simulink model "Milford"  (R2017a)
settings: Solver=FixedStepAuto  StartTime=0.0  StopTime=Cycle_End  FixedStep=0.01  MaxStep=0.01  RelTol=1e-3  EnableMultiTasking=on
PostLoadFcn:
  | , if any(exist('dsrtsu_mdlpostloadfcn', 'file') == [2, 3, 6]), try dsrtsu_mdlpostloadfcn('Execute', bdroot); catch fprintf('Error in PostLoadFcn (dsrtsu_mdlpostloadfcn) for model "%s":\n %s\n', bdroot, lasterr); end, end,
undefined symbols (not defined in the file): Actuators, APP1_OOR, APP2_OOR, APP_Mismatch, Brk_Flt, cal, ClutchEngag, DiscIntNeverNeededParam, eng, Engine, EngOverTemp, ENGTRQ_MSMCH_Degraded_CP, ENGTRQ_MSMCH_ErrCritical_CP, ENGTRQ_MSMCH_LimpHome_CP, EngTrqMismatch, ESSOverTemp, gb, Gearbox, KeyPos_Flt, lib_Actuators, lib_Sensors_2017a, lib_Transmission, Loss, LossCAN, MCUOverTemp, mot, MotDirMismatch, MotOverTemp, MotTrqMismatch, mph2kph, PRNDL_Flt, Ratio, RegenFault, Sensors, Spd, time, Transmission
libraries: simulink x110, powerlib_meascontrol x6, EC2_libraries x5, dspsigops x3, lib_Chassis x1, lib_DCDC x1, lib_Differential x1, lib_HVESS x1, lib_Engine x1, lib_OBC x1, Transmission_Validation x1, lib_Wheels x1
(part 4 of 9)

== system Milford/Controller_with_Transmission_Manager1/HSC/Driver_Requests/APP_BPP to DrvIntndAxlTrq2/Post Driver Intnded Axle Torque ==
  note: //*mode==1 (CD Mode)
      | mode==2 (CS Mode - Engine Drive)
      | mode==3 (CS Mode-Motor Drive) pass MotTrq
      | mode==4 (Sports Mode) pass Mot Trq+Eng Trq
      | mode==5 (Engine only mode)*//
  APP : Inport
  BPP : Inport  Port=2
  VehicleSpeed : Inport  Port=3
  TransGearRatio : Inport  Port=4
  Mode : Inport  Port=5
  Motor_Speed : Inport  Port=6
  APP1 : InportShadow
  Abs : Abs
  Add : Sum
  Brake Command : Subsystem
  Bus Creator1 : BusCreator  Inputs=1
  Bus Creator3 : BusCreator  Inputs=3
  Driver Intended Axle Torque : Subsystem
  Switch : Switch  Threshold=cal.Regen.MinMotSpd
  rad/s to RPM2 : Gain  Gain=30/pi
  IntndAxlTrq : Outport
  BrkIntndAxlTrq : Outport  Port=2
  tag scope: DrvIntdAxleTrq=global
  wires:
  APP/1 -> Brake Command/1(APP)
  Driver Intended Axle Torque/1(DrvIntndAxlTrq) -> Add/1, [DrvIntdAxleTrq]  "DrvIntndAxlTrq"
  BPP/1 -> Brake Command/2(BPP)
  VehicleSpeed/1 -> Brake Command/3(VehicleSpeed)
  Mode/1 -> Driver Intended Axle Torque/2(Mode)
  TransGearRatio/1 -> Driver Intended Axle Torque/3(TransGearRatio)
  Brake Command/1(BrkAxlTrq) -> Add/2, Bus Creator1/1, Bus Creator3/3  "BrkIntndAxlTrq"
  Bus Creator1/1 -> BrkIntndAxlTrq/1
  Motor_Speed/1 -> rad/s to RPM2/1
  Abs/1 -> Switch/2
  Add/1 -> Switch/1  "FullDrvIntndAxlTrq"
  Switch/1 -> Bus Creator3/1  "FullDrvIntndAxlTrq"
  Bus Creator3/1 -> IntndAxlTrq/1  "IntndAxlTrq"
  [DrvIntdAxleTrq] -> Bus Creator3/2
  APP1/1 -> Driver Intended Axle Torque/1(APP)
  [DrvIntdAxleTrq] -> Switch/3
  rad/s to RPM2/1 -> Abs/1

== system Milford/Controller_with_Transmission_Manager1/HSC/Powertrain Manager/HV Manager/Axiomatic_Output_Manager ==
  Sensors : Inport
  HV_Bus_Status : Inport  Port=2
  Bus Creator : BusCreator  Inputs=3
  Bus Selector : BusSelector  OutputSignals=GFD_Light
  Bus Selector1 : BusSelector  OutputSignals=from_CAN.fromHV_CAN.from_OBC.NLG5_ST.NLG5_S_CP_DT,from_CAN.fromEBCAN.from_ECM.EngRunAtv
  Compare To Constant1 : simulink/Logic and Bit Operations/Compare To Constant  relop===  const=1  OutDataTypeStr=boolean
  Data Type Conversion : DataTypeConversion
  Logical Operator : Logic  AllPortsSameDT=off  OutDataTypeStr=boolean
  Logical Operator1 : Logic  Operator=NOT  AllPortsSameDT=off  OutDataTypeStr=boolean
  Axiomatic_CAN : Outport
  wires:
  [HV_Charge_Indicator] -> Data Type Conversion/1
  Sensors/1 -> Bus Selector1/1
  Logical Operator/1 -> Bus Creator/3  "Veh_Ready_Light"
  Data Type Conversion/1 -> Bus Creator/2  "HV_Chg_Light"
  Bus Selector/1 -> Bus Creator/1  "<GFD_Light>"
  Bus Creator/1 -> Axiomatic_CAN/1  "Axiomatic_CAN"
  HV_Bus_Status/1 -> Bus Selector/1
  Compare To Constant1/1 -> Logical Operator/2
  Logical Operator1/1 -> Logical Operator/1
  Bus Selector1/2 -> Compare To Constant1/1  "<EngRunAtv>"
  Bus Selector1/1 -> Logical Operator1/1  "<NLG5_S_CP_DT>"

== system Milford/Controller_with_Transmission_Manager1/HSC/Powertrain Manager/HV Manager/BMS_Manager ==
  note: Control Pilot signal added 02/14/2017
      | to charge automatically
  Sensors : Inport
  Controls : Inport  Port=2
  Bus Creator : BusCreator  Inputs=3
  Bus Creator1 : BusCreator  Inputs=8
  Bus Creator2 : BusCreator  Inputs=2
  Bus Creator3 : BusCreator  Inputs=6
  Bus Creator4 : BusCreator  Inputs=5
  Bus Selector : BusSelector  OutputSignals=closeMaincReq
  Bus Selector1 : BusSelector  OutputSignals=from_CAN.fromHV_CAN.from_BMSHybrid.BMS_HYB_02.BMS_Fehler_HS_offen,from_CAN.fromHV_CAN.from_BMSHybrid.BMS_HYB_02.BMS_Fehler_Pilot,from_CAN.fromHV_CAN.from_BMSHybrid.BMS_HYB_02.BMS_Init_abgeschlossen,from_CAN.fromHV_CAN.from_BMSHybrid.BMS_HYB_02.BMS_IstModus,from_CAN.fromHV_CAN.from_BMSHybrid.BMS_HYB_02.BMS_IstSpannung,from_CAN.fromHV_CAN.from_BMSHybrid.BMS_HYB_02.BMS_IstStrom,from_CAN.fromHV_CAN.from_BMSHybrid.BMS_HYB_02.BMS_SleepInd
  Bus Selector2 : BusSelector  OutputSignals=from_CAN.fromEBCAN.from_BMSAntrieb.NMH_BMS.NMH_BMS_Car_WakeUp,from_CAN.fromEBCAN.from_BMSAntrieb.NMH_BMS.NMH_BMS_Normal_Mode_1,from_CAN.fromEBCAN.from_BMSAntrieb.NMH_BMS.NMH_BMS_Normal_Mode_2,from_CAN.fromEBCAN.from_BMSAntrieb.NMH_BMS.NMH_BMS_Start_1,from_CAN.fromEBCAN.from_BMSAntrieb.NMH_BMS.NMH_BMS_Start_2,from_CAN.fromVEH_CAN.from_BCM.SysPwrMd,from_CAN.fromEBCAN.from_ECM.EngRunAtv
  Bus Selector3 : BusSelector  OutputSignals=from_CAN.fromHV_CAN.from_BMSHybrid.BMS_Spannung_ZwKr
  Bus Selector4 : BusSelector  OutputSignals=HV_req
  Bus Selector5 : BusSelector  OutputSignals=from_CAN.fromHV_CAN.from_OBC.NLG5_ST.NLG5_S_CP_DT
  Controls1 : InportShadow  Port=2
  Data Type Conversion{,1,6..8} (5 alike) : DataTypeConversion  OutDataTypeStr=boolean
  ESS_Manager : Stateflow chart  TreatAsAtomicUnit=on
  Edge Detector : powerlib_meascontrol/Logic/Edge Detector  model=Either  ic=0  Ts=0
      settings: SourceProductName=Simscape Power Systems  SourceProductBaseCode=PS
  Fault Latch : Subsystem
  ISO_Hybrid_01_Req : Subsystem
  Isolation Fault Calculation : Subsystem
  BMS CAN : Outport
  HV_BUS_Status : Outport  Port=2
  BMS Digital : Outport  Port=3
  wires:
  ISO_Hybrid_01_Req/1(Out1) -> Bus Creator/2
  ESS_Manager/9(ISO_Hybrid_01_Req) -> ISO_Hybrid_01_Req/1(In1)
  ESS_Manager/11(MO_BMS_Sollmodus) -> Bus Creator2/2
  Sensors/1 -> Bus Selector2/1, Bus Selector3/1, Isolation Fault Calculation/1(Sensors1), Bus Selector5/1, Bus Selector1/1
  Data Type Conversion1/1 -> Bus Creator4/5  "chg_wake"
  Bus Creator4/1 -> BMS Digital/1  "BMS_Digital"
  Bus Creator/1 -> BMS CAN/1  "BMS_CAN"
  Controls1/1 -> Bus Selector4/1
  Bus Selector/1 -> ESS_Manager/19(closeMaincReq)  "<closeMaincReq>"
  Controls/1 -> Bus Selector/1
  Bus Creator3/1 -> HV_BUS_Status/1  "HV_BUS_Status"
  ESS_Manager/18(HV_State) -> Bus Creator3/2
  ESS_Manager/15(veh_wake) -> Bus Creator4/4
  ESS_Manager/14(T_30C) -> Bus Creator4/3
  ESS_Manager/16(chga_wake) -> Data Type Conversion1/1
  ESS_Manager/13(T_30) -> Bus Creator4/2
  ESS_Manager/21(Shutdown_Complete) -> Bus Creator3/5
  ESS_Manager/20(ReadyToCharge) -> Data Type Conversion7/1
  ESS_Manager/19(ReadyToDrive) -> Data Type Conversion6/1
  ESS_Manager/17(HVDischarge) -> Data Type Conversion8/1
  Bus Creator1/1 -> Bus Creator/1  "ISO_Funktionaler_Req_All"
  Data Type Conversion8/1 -> Bus Creator3/1  "HV Discharge"
  Data Type Conversion7/1 -> Bus Creator3/4  "ReadyToCharge"
  Data Type Conversion6/1 -> Bus Creator3/3  "ReadyToDrive"
  ESS_Manager/12(T_15) -> Bus Creator4/1
  ESS_Manager/10(MO_SleepAckn) -> Bus Creator2/1
  ESS_Manager/8(Diag_Rq_Fktnl_Data_OBD_byte_7) -> Bus Creator1/8
  ESS_Manager/7(Diag_Rq_Fktnl_Data_OBD_byte_6) -> Bus Creator1/7
  ESS_Manager/6(Diag_Rq_Fktnl_Data_OBD_byte_5) -> Bus Creator1/6
  ESS_Manager/5(Diag_Rq_Fktnl_Data_OBD_byte_4) -> Bus Creator1/5
  ESS_Manager/4(Diag_Rq_Fktnl_Data_OBD_byte_3) -> Bus Creator1/4
  ESS_Manager/3(Diag_Rq_Fktnl_Data_OBD_byte_2) -> Bus Creator1/3
  ESS_Manager/2(Diag_Rq_Fktnl_Data_OBD_byte_1) -> Bus Creator1/2
  ESS_Manager/1(Diag_Rq_Fktnl_Data_OBD_byte_0) -> Bus Creator1/1
  Bus Selector5/1 -> Data Type Conversion/1  "<NLG5_S_CP_DT>"
  Bus Selector3/1 -> ESS_Manager/11(BMS_Spannung_ZwKr)  "<BMS_Spannung_ZwKr>"
  Bus Selector2/3 -> ESS_Manager/14(NMH_BMS_Normal_Mode_2)  "<NMH_BMS_Normal_Mode_2>"
  Bus Selector2/2 -> ESS_Manager/13(NMH_Normal_Mode_1)  "<NMH_BMS_Normal_Mode_1>"
  Bus Selector2/1 -> ESS_Manager/12(NMH_BMS_Car_WakeUp)  "<NMH_BMS_Car_WakeUp>"
  Bus Selector1/5 -> ESS_Manager/7(BMS_IstSpannung)  "<BMS_IstSpannung>"
  Bus Selector1/4 -> ESS_Manager/6(BMS_IstModus)  "<BMS_IstModus>"
  Bus Selector1/3 -> ESS_Manager/5(BMS_Init_abgeschlossen)  "<BMS_Init_abgeschlossen>"
  Bus Selector1/2 -> ESS_Manager/4(BMS_Fehler_Pilot)  "<BMS_Fehler_Pilot>"
  Bus Selector1/1 -> ESS_Manager/3(BMS_Fehler_HS_offen)  "<BMS_Fehler_HS_offen>"
  Isolation Fault Calculation/1(IsoFault) -> Fault Latch/1(IsoFault)
  Fault Latch/1(IsoFaultLatched) -> ESS_Manager/1(ISOfault)
  Bus Creator2/1 -> Bus Creator/3  "MSG_HYB_01"
  Bus Selector4/1 -> ESS_Manager/10(HV_req)  "<HV_req>"
  Bus Selector2/6 -> Edge Detector/1  "<SysPwrMd>"
  Edge Detector/1 -> ESS_Manager/17(KeyPos)
  Bus Selector2/7 -> ESS_Manager/18(EngRunAtv)  "<EngRunAtv>"
  Bus Selector2/5 -> ESS_Manager/16(NMH_BMS_Start_2)  "<NMH_BMS_Start_2>"
  Bus Selector2/4 -> ESS_Manager/15(NMH_BMS_Start_1)  "<NMH_BMS_Start_1>"
  Bus Selector1/7 -> ESS_Manager/9(BMS_SleepInd)  "<BMS_SleepInd>"
  Bus Selector1/6 -> ESS_Manager/8(BMS_IstStrom)  "<BMS_IstStrom>"
  Data Type Conversion/1 -> ESS_Manager/2(plugged)
  ESS_Manager/22(GFD_Light) -> Bus Creator3/6  "GFD_Light"

== system Milford/Controller_with_Transmission_Manager1/HSC/Powertrain Manager/HV Manager/DCDC Manager ==
  BMSInput : Inport
  Control : Inport  Port=2
  Bus Creator : BusCreator  Inputs=6
  Bus Selector : BusSelector  OutputSignals=from_CAN.fromHV_CAN.from_MCU.INV_VCU_01.INV_State
  Bus Selector1 : BusSelector  OutputSignals=from_CAN.fromHV_CAN.from_BMSHybrid.BMS_HYB_02.BMS_IstSpannung,from_CAN.fromHV_CAN.from_BMSHybrid.BMS_Spannung_ZwKr,from_CAN.fromHV_CAN.from_BMSHybrid.BMS_HYB_02.BMS_Fehler_Pilot
  Bus Selector2 : BusSelector  OutputSignals=mode,powerMode
  Contactors status check : Subsystem
  DCDCManager : Stateflow chart  RequirementInfo={} %GIDa_e7a9563c_45c2_4f7a_81ef_fb4c6797264a  TreatAsAtomicUnit=on
  DCModeOverride : Subsystem
  DCDC_Status : Outport
  wires:
  BMSInput/1 -> Bus Selector/1, Bus Selector1/1
  Bus Selector1/1 -> Contactors status check/1(BMS_Voltage)  "<BMS_IstSpannung>"
  Bus Selector1/3 -> Contactors status check/3(BMS_HVILfault)  "<BMS_Fehler_Pilot>"
  Bus Selector1/2 -> Contactors status check/2(BMS_LinkVoltage)  "<BMS_Spannung_ZwKr>"
  Contactors status check/1(Out1) -> DCDCManager/1(ContactorsFailed)  "ContactorsFailed"
  Bus Selector/1 -> DCDCManager/2(INV_state)  "<INV_State>"
  DCDCManager/5(CurrentLV) -> Bus Creator/5  "CurrentLV"
  DCDCManager/4(VoltageLV) -> Bus Creator/4  "VoltageLV"
  DCDCManager/3(CurrentHV) -> Bus Creator/3  "CurrentHV"
  DCDCManager/2(VoltageHV) -> Bus Creator/2  "VoltageHV"
  Bus Creator/1 -> DCDC_Status/1  "DCDC_Out"
  DCDCManager/6(DCDC_State) -> Bus Creator/6  "DCDC_State"
  Bus Selector2/1 -> DCDCManager/3(mode)  "<mode>"
  Control/1 -> Bus Selector2/1
  Bus Selector2/2 -> DCDCManager/4(powerMode)  "<powerMode>"
  DCDCManager/1(DCmode) -> DCModeOverride/1(In1)  "DC_mode"
  DCModeOverride/1(Out1) -> Bus Creator/1

== system Milford/Controller_with_Transmission_Manager1/HSC/Powertrain Manager/HV Manager/Inverter Manager ==
  HV_Bus_Status : Inport
  Sensors : Inport  Port=2
  Control : Inport  Port=3
  Bus Creator2 : BusCreator  Inputs=1
  Bus Creator3 : BusCreator  Inputs=2
  Bus Creator4 : BusCreator  Inputs=1
  Bus Creator5 : BusCreator  Inputs=1
  Bus Selector : BusSelector  OutputSignals=ReadyToDrive,ReadyToCharge
  Bus Selector1 : BusSelector  OutputSignals=EnableInverter
  Bus Selector3 : BusSelector  OutputSignals=from_CAN.fromHV_CAN.from_MCU.INV_VCU_01.MessageCounter,from_CAN.fromHV_CAN.from_MCU.INV_VCU_01.INV_State,from_CAN.fromHV_CAN.from_MCU.INV_VCU_01.INV_CurrentHV
  Data Type Conversion : DataTypeConversion  OutDataTypeStr=boolean
  Data Type Conversion1 : DataTypeConversion  OutDataTypeStr=boolean
  Data Type Conversion2 : DataTypeConversion
  Data Type Conversion3 : DataTypeConversion  OutDataTypeStr=boolean
  Detect Change1 : simulink/Logic and Bit Operations/Detect Change  vinit=0  OutDataTypeStr=boolean
  HVCAN_State : Constant
  "MCU_Manager " : Stateflow chart  RequirementInfo={} %GIDa_b24a457d_d0fa_492f_a0c6_5192198f8f6c  TreatAsAtomicUnit=on
  RequestOverride : Subsystem
  ShutdownCurrent : Constant  Value=0.5
  MCU_Status : Outport
  MCU_CAN : Outport  Port=2
  MCU_Torque_disconnect : Outport  Port=3
  MCU_Relay : Outport  Port=4
  wires:
  HVCAN_State/1 -> Data Type Conversion2/1  "HVCAN_State"
  Bus Selector3/1 -> Detect Change1/1  "<MessageCounter>"
  Bus Selector3/2 -> "MCU_Manager "/5(INV_State)  "<INV_State>"
  Data Type Conversion1/1 -> "MCU_Manager "/7(EnableInverter)
  Data Type Conversion/1 -> "MCU_Manager "/1(ReadyToDrive)
  Bus Creator5/1 -> MCU_Torque_disconnect/1
  "MCU_Manager "/2(Motor_Torque_Command) -> Bus Creator5/1  "Motor_Torque_Command"
  Bus Creator4/1 -> MCU_Relay/1
  "MCU_Manager "/3(INVCON_Power) -> Bus Creator4/1  "INVCON_Power"
  Bus Creator2/1 -> MCU_Status/1
  "MCU_Manager "/1(MCU_State) -> Bus Creator2/1  "MCU_State"
  Bus Selector3/3 -> "MCU_Manager "/6(INV_CurrentHV)  "<INV_CurrentHV>"
  ShutdownCurrent/1 -> "MCU_Manager "/8(ShutdownCurrent)  "ShutdownCurrent"
  Bus Selector/1 -> Data Type Conversion/1  "<ReadyToDrive>"
  HV_Bus_Status/1 -> Bus Selector/1  "HV_Bus Status"
  Bus Selector1/1 -> Data Type Conversion1/1  "<EnableInverter>"
  Sensors/1 -> Bus Selector3/1  "Sensors"
  Bus Creator3/1 -> MCU_CAN/1
  Data Type Conversion2/1 -> "MCU_Manager "/3(HVCAN_State)  "HVCAN_State"
  Bus Selector/2 -> Data Type Conversion3/1  "<ReadyToCharge>"
  Data Type Conversion3/1 -> "MCU_Manager "/2(ReadyToCharge)
  Detect Change1/1 -> "MCU_Manager "/4(INVCON_Power_Feedback)  "INVCON_Power_Feedback"
  "MCU_Manager "/5(CAN_Activation) -> Bus Creator3/2  "VCU_flgInvrCanActvnCmd"
  Control/1 -> Bus Selector1/1
  "MCU_Manager "/4(RequestedStateINV) -> RequestOverride/1(In1)  "VCU_RequestedStateINVOut"
  RequestOverride/1(Out1) -> Bus Creator3/1

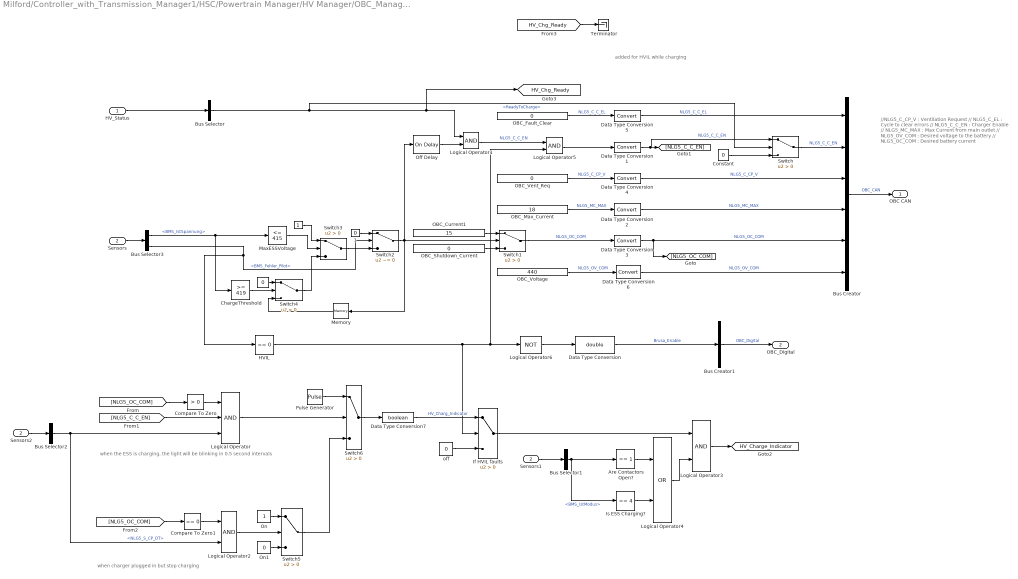
== system Milford/Controller_with_Transmission_Manager1/HSC/Powertrain Manager/HV Manager/OBC_Manager ==
  note: added for HVIL
      | while charging
  note: //NLG5_C_CP_V : Ventilation Request
      | // NLG5_C_EL : Cycle to clear errors
      | // NLG5_C_C_EN : Charger Enable
      | // NLG5_MC_MAX : Max Current from main outlet
      | // NLG5_OV_COM : Desired voltage to the battery
      | // NLG5_OC_COM : Desired battery current
  note: when charger plugged in but stop charging
  note: when the ESS is charging, the light will be blinking in 0.5 second intervals
  HV_Status : Inport
  Sensors : Inport  Port=2
  " " : Constant
  "   " : Constant  Value=0
  "   1" : Constant  Value=0
  Are Contactors Open? : simulink/Logic and Bit Operations/Compare To Constant  relop===  const=1  OutDataTypeStr=boolean
  Bus Creator : BusCreator  Inputs=6
  Bus Creator1 : BusCreator  Inputs=1
  Bus Selector : BusSelector  OutputSignals=ReadyToCharge
  Bus Selector1 : BusSelector  OutputSignals=from_CAN.fromHV_CAN.from_BMSHybrid.BMS_HYB_02.BMS_IstModus
  Bus Selector2 : BusSelector  OutputSignals=from_CAN.fromHV_CAN.from_OBC.NLG5_ST.NLG5_S_CP_DT
  Bus Selector3 : BusSelector  OutputSignals=from_CAN.fromHV_CAN.from_BMSHybrid.BMS_HYB_02.BMS_IstSpannung,from_CAN.fromHV_CAN.from_BMSHybrid.BMS_HYB_02.BMS_Fehler_Pilot
  ChargeThreshold : simulink/Logic and Bit Operations/Compare To Constant  relop=>=  const=419  OutDataTypeStr=boolean
  Compare To Zero : simulink/Logic and Bit Operations/Compare To Zero  relop=>  OutDataTypeStr=boolean
  Compare To Zero1 : simulink/Logic and Bit Operations/Compare To Zero  relop===  OutDataTypeStr=boolean
  Constant : Constant  Value=0
  Data Type Conversion : DataTypeConversion  OutDataTypeStr=double
  Data Type Conversion{1..6} (6 alike) : DataTypeConversion
  Data Type Conversion7 : DataTypeConversion  OutDataTypeStr=boolean
  HVIL : simulink/Logic and Bit Operations/Compare To Constant  relop===  const=0  OutDataTypeStr=boolean
  If HVIL faults : Switch  Criteria=u2 > Threshold
  Is ESS Charging? : simulink/Logic and Bit Operations/Compare To Constant  relop===  const=4  OutDataTypeStr=boolean
  Logical Operator : Logic  Inputs=3  AllPortsSameDT=off  OutDataTypeStr=boolean
  Logical Operator{1..3,5} (4 alike) : Logic  AllPortsSameDT=off  OutDataTypeStr=boolean
  Logical Operator4 : Logic  Operator=OR  AllPortsSameDT=off  OutDataTypeStr=boolean
  Logical Operator6 : Logic  Operator=NOT  Inputs=3  AllPortsSameDT=off  OutDataTypeStr=boolean
  MaxESSVoltage : simulink/Logic and Bit Operations/Compare To Constant  relop=<=  const=415  OutDataTypeStr=boolean
  Memory : Memory  InheritSampleTime=on
  OBC_Current1 : Constant  Value=15
  OBC_Fault_Clear : Constant  Value=0
  OBC_Max_Current : Constant  Value=18
  OBC_Shutdown_Current : Constant  Value=0
  OBC_Vent_Req : Constant  Value=0
  OBC_Voltage : Constant  Value=440
  Off Delay : powerlib_meascontrol/Logic/On Delay  DelayType=Off delay  delay=30  ic=0  Ts=0
      settings: SourceProductName=Simscape Power Systems
  On : Constant
  On1 : Constant  Value=0
  Pulse Generator : DiscretePulseGenerator  PulseType=Time based  Period=1  PulseWidth=50
  Sensors1 : InportShadow  Port=2
  Sensors2 : InportShadow  Port=2
  Switch{,1,3..6} (6 alike) : Switch  Criteria=u2 > Threshold
  Switch2 : Switch  Criteria=u2 ~= 0
  Terminator : Terminator
  off : Constant  Value=0
  OBC CAN : Outport
  OBC_Digital : Outport  Port=2
  tag scope: HV_Charge_Indicator=global, HV_Chg_Ready=global
  wires:
  Data Type Conversion7/1 -> If HVIL faults/1  "HV_Charg_Indicator"
  OBC_Voltage/1 -> Data Type Conversion6/1  "NLG5_OV_COM"
  OBC_Max_Current/1 -> Data Type Conversion2/1  "NLG5_MC_MAX"
  OBC_Fault_Clear/1 -> Data Type Conversion5/1  "NLG5_C_C_EL"
  OBC_Vent_Req/1 -> Data Type Conversion4/1  "NLG5_C_CP_V"
  Switch1/1 -> Data Type Conversion3/1  "NLG5_OC_COM"
  Logical Operator1/1 -> Logical Operator5/1  "NLG5_C_C_EN"
  Data Type Conversion1/1 -> Switch/1, [NLG5_C_C_EN]  "NLG5_C_C_EN"
  Switch4/1 -> Switch3/3
  Memory/1 -> Switch4/3
  OBC_Shutdown_Current/1 -> Switch1/3
  " "/1 -> Switch3/1
  ChargeThreshold/1 -> Switch4/2
  "   "/1 -> Switch4/1
  Switch2/1 -> Memory/1, Off Delay/1, Switch1/2
  OBC_Current1/1 -> Switch1/1
  Data Type Conversion3/1 -> Bus Creator/5, [NLG5_OC_COM]  "NLG5_OC_COM"
  Data Type Conversion6/1 -> Bus Creator/6  "NLG5_OV_COM"
  Data Type Conversion4/1 -> Bus Creator/3  "NLG5_C_CP_V"
  Data Type Conversion5/1 -> Bus Creator/1  "NLG5_C_C_EL"
  Data Type Conversion2/1 -> Bus Creator/4  "NLG5_MC_MAX"
  Bus Selector3/1 -> ChargeThreshold/1, MaxESSVoltage/1  "<BMS_IstSpannung>"
  Off Delay/1 -> Logical Operator1/2
  Bus Selector/1 -> Switch/2, Logical Operator1/1, [HV_Chg_Ready]  "<ReadyToCharge>"
  MaxESSVoltage/1 -> Switch3/2
  HV_Status/1 -> Bus Selector/1
  Bus Creator/1 -> OBC CAN/1  "OBC_CAN"
  Sensors/1 -> Bus Selector3/1
  [NLG5_OC_COM] -> Compare To Zero/1
  Compare To Zero/1 -> Logical Operator/1
  [NLG5_C_C_EN] -> Logical Operator/2
  Logical Operator/1 -> Switch6/2
  Pulse Generator/1 -> Switch6/1
  [NLG5_OC_COM] -> Compare To Zero1/1
  Compare To Zero1/1 -> Logical Operator2/1
  Logical Operator2/1 -> Switch5/2
  On/1 -> Switch5/1
  On1/1 -> Switch5/3
  Switch5/1 -> Switch6/3
  Switch6/1 -> Data Type Conversion7/1
  Bus Selector3/2 -> HVIL/1, Switch2/2  "<BMS_Fehler_Pilot>"
  Data Type Conversion/1 -> Bus Creator1/1  "Brusa_Enable"
  Bus Creator1/1 -> OBC_Digital/1  "OBC_Digital"
  Switch3/1 -> Switch2/3
  "   1"/1 -> Switch2/1
  HVIL/1 -> Logical Operator5/2, Logical Operator6/1, If HVIL faults/2
  If HVIL faults/1 -> Logical Operator3/1
  off/1 -> If HVIL faults/3
  Logical Operator3/1 -> [HV_Charge_Indicator]
  Sensors1/1 -> Bus Selector1/1
  Are Contactors Open?/1 -> Logical Operator4/1
  Bus Selector1/1 -> Is ESS Charging?/1, Are Contactors Open?/1  "<BMS_IstModus>"
  Is ESS Charging?/1 -> Logical Operator4/2
  Logical Operator4/1 -> Logical Operator3/2
  Logical Operator5/1 -> Data Type Conversion1/1
  Logical Operator6/1 -> Data Type Conversion/1
  Constant/1 -> Switch/3
  Switch/1 -> Bus Creator/2  "NLG5_C_C_EN"
  Sensors2/1 -> Bus Selector2/1
  Bus Selector2/1 -> Logical Operator2/2, Logical Operator/3  "<NLG5_S_CP_DT>"
  [HV_Chg_Ready] -> Terminator/1

== system Milford/Controller_with_Transmission_Manager1/HSC/Powertrain Manager/HV Manager1/Axiomatic_Output_Manager ==
  Sensors : Inport
  HV_Bus_Status : Inport  Port=2
  Bus Creator : BusCreator  Inputs=3
  Bus Selector : BusSelector  OutputSignals=GFD_Light
  Bus Selector1 : BusSelector  OutputSignals=from_CAN.fromEBCAN.from_ECM.EngRunAtv
  Bus Selector5 : BusSelector  OutputSignals=from_CAN.fromHV_CAN.from_OBC.NLG5_ST.NLG5_S_CP_DT
  Compare To Constant1 : simulink/Logic and Bit Operations/Compare To Constant  relop===  const=1  OutDataTypeStr=boolean
      link override Compare: Operator===  OutDataTypeStr=boolean
  Data Type Conversion : DataTypeConversion
  Logical Operator : Logic  AllPortsSameDT=off  OutDataTypeStr=boolean
  Logical Operator1 : Logic  Operator=NOT  AllPortsSameDT=off  OutDataTypeStr=boolean
  Sensors1 : InportShadow
  Axiomatic_CAN : Outport
  wires:
  Sensors1/1 -> Bus Selector5/1
  Bus Selector1/1 -> Compare To Constant1/1  "<EngRunAtv>"
  Bus Selector5/1 -> Logical Operator1/1  "<NLG5_S_CP_DT>"
  Logical Operator1/1 -> Logical Operator/1
  Compare To Constant1/1 -> Logical Operator/2
  HV_Bus_Status/1 -> Bus Selector/1
  Bus Creator/1 -> Axiomatic_CAN/1  "Axiomatic_CAN"
  Bus Selector/1 -> Bus Creator/1  "<GFD_Light>"
  Data Type Conversion/1 -> Bus Creator/2  "HV_Chg_Light"
  Logical Operator/1 -> Bus Creator/3  "Veh_Ready_Light"
  Sensors/1 -> Bus Selector1/1
  [HV_Charge_Indicator] -> Data Type Conversion/1

== system Milford/Controller_with_Transmission_Manager1/HSC/Powertrain Manager/HV Manager1/BMS_Manager ==
  note: Control Pilot signal added 02/14/2017
      | to charge automatically
  Sensors : Inport
  Controls : Inport  Port=2
  In1 : Inport  Port=3
  Bus Creator : BusCreator  Inputs=3
  Bus Creator1 : BusCreator  Inputs=8
  Bus Creator2 : BusCreator  Inputs=2
  Bus Creator3 : BusCreator  Inputs=6
  Bus Creator4 : BusCreator  Inputs=5
  Bus Selector : BusSelector  OutputSignals=closeMaincReq
  Bus Selector1 : BusSelector  OutputSignals=from_CAN.fromHV_CAN.from_BMSHybrid.BMS_HYB_02.BMS_Fehler_HS_offen,from_CAN.fromHV_CAN.from_BMSHybrid.BMS_HYB_02.BMS_Fehler_Pilot,from_CAN.fromHV_CAN.from_BMSHybrid.BMS_HYB_02.BMS_Init_abgeschlossen,from_CAN.fromHV_CAN.from_BMSHybrid.BMS_HYB_02.BMS_IstModus,from_CAN.fromHV_CAN.from_BMSHybrid.BMS_HYB_02.BMS_IstSpannung,from_CAN.fromHV_CAN.from_BMSHybrid.BMS_HYB_02.BMS_IstStrom,from_CAN.fromHV_CAN.from_BMSHybrid.BMS_HYB_02.BMS_SleepInd
  Bus Selector2 : BusSelector  OutputSignals=from_CAN.fromEBCAN.from_BMSAntrieb.NMH_BMS.NMH_BMS_Car_WakeUp,from_CAN.fromEBCAN.from_BMSAntrieb.NMH_BMS.NMH_BMS_Normal_Mode_1,from_CAN.fromEBCAN.from_BMSAntrieb.NMH_BMS.NMH_BMS_Normal_Mode_2,from_CAN.fromEBCAN.from_BMSAntrieb.NMH_BMS.NMH_BMS_Start_1,from_CAN.fromEBCAN.from_BMSAntrieb.NMH_BMS.NMH_BMS_Start_2,from_CAN.fromVEH_CAN.from_BCM.SysPwrMd,from_CAN.fromEBCAN.from_ECM.EngRunAtv
  Bus Selector3 : BusSelector  OutputSignals=from_CAN.fromHV_CAN.from_BMSHybrid.BMS_Spannung_ZwKr
  Bus Selector4 : BusSelector  OutputSignals=HV_req
  Bus Selector5 : BusSelector  OutputSignals=from_CAN.fromHV_CAN.from_OBC.NLG5_ST.NLG5_S_CP_DT
  Bus Selector7 : BusSelector  OutputSignals=DCDC_State
  Constant : Constant  Value=3
  Controls1 : InportShadow  Port=2
  Data Type Conversion{,1,6..8} (5 alike) : DataTypeConversion  OutDataTypeStr=boolean
  ESS_Manager : Stateflow chart  TreatAsAtomicUnit=on
  Edge Detector : powerlib_meascontrol/Logic/Edge Detector  model=Either  ic=0  Ts=0
      settings: SourceProductName=Simscape Power Systems  SourceProductBaseCode=PS
  Fault Latch : Subsystem
  GFD_OvrrdSwitch : Constant  Value=0
  GFD_OvrrdValue : Constant
  ISO_Hybrid_01_Req : Subsystem
  Isolation Fault Calculation : Subsystem
  Switch : Switch  Criteria=u2 > Threshold
  BMS CAN : Outport
  HV_BUS_Status : Outport  Port=2
  BMS Digital : Outport  Port=3
  wires:
  Bus Selector7/1 -> ESS_Manager/21(DCDC_State)  "<DCDC_State>"
  In1/1 -> Bus Selector7/1
  Constant/1 -> ESS_Manager/20(INV_State)
  GFD_OvrrdValue/1 -> Switch/1
  GFD_OvrrdSwitch/1 -> Switch/2
  ESS_Manager/22(GFD_Light) -> Switch/3  "GFD_Light"
  Data Type Conversion/1 -> ESS_Manager/2(plugged)
  Bus Selector1/6 -> ESS_Manager/8(BMS_IstStrom)  "<BMS_IstStrom>"
  Bus Selector1/7 -> ESS_Manager/9(BMS_SleepInd)  "<BMS_SleepInd>"
  Bus Selector2/4 -> ESS_Manager/15(NMH_BMS_Start_1)  "<NMH_BMS_Start_1>"
  Bus Selector2/5 -> ESS_Manager/16(NMH_BMS_Start_2)  "<NMH_BMS_Start_2>"
  Bus Selector2/7 -> ESS_Manager/18(EngRunAtv)  "<EngRunAtv>"
  Edge Detector/1 -> ESS_Manager/17(KeyPos)
  Bus Selector2/6 -> Edge Detector/1  "<SysPwrMd>"
  Bus Selector4/1 -> ESS_Manager/10(HV_req)  "<HV_req>"
  Bus Creator2/1 -> Bus Creator/3  "MSG_HYB_01"
  Fault Latch/1(IsoFaultLatched) -> ESS_Manager/1(ISOfault)
  Isolation Fault Calculation/1(IsoFault) -> Fault Latch/1(IsoFault)
  Switch/1 -> Bus Creator3/6  "GFD_Light"
  Bus Selector1/1 -> ESS_Manager/3(BMS_Fehler_HS_offen)  "<BMS_Fehler_HS_offen>"
  Bus Selector1/2 -> ESS_Manager/4(BMS_Fehler_Pilot)  "<BMS_Fehler_Pilot>"
  Bus Selector1/3 -> ESS_Manager/5(BMS_Init_abgeschlossen)  "<BMS_Init_abgeschlossen>"
  Bus Selector1/4 -> ESS_Manager/6(BMS_IstModus)  "<BMS_IstModus>"
  Bus Selector1/5 -> ESS_Manager/7(BMS_IstSpannung)  "<BMS_IstSpannung>"
  Bus Selector2/1 -> ESS_Manager/12(NMH_BMS_Car_WakeUp)  "<NMH_BMS_Car_WakeUp>"
  Bus Selector2/2 -> ESS_Manager/13(NMH_Normal_Mode_1)  "<NMH_BMS_Normal_Mode_1>"
  Bus Selector2/3 -> ESS_Manager/14(NMH_BMS_Normal_Mode_2)  "<NMH_BMS_Normal_Mode_2>"
  Bus Selector3/1 -> ESS_Manager/11(BMS_Spannung_ZwKr)  "<BMS_Spannung_ZwKr>"
  Bus Selector5/1 -> Data Type Conversion/1  "<NLG5_S_CP_DT>"
  ESS_Manager/1(Diag_Rq_Fktnl_Data_OBD_byte_0) -> Bus Creator1/1
  ESS_Manager/2(Diag_Rq_Fktnl_Data_OBD_byte_1) -> Bus Creator1/2
  ESS_Manager/3(Diag_Rq_Fktnl_Data_OBD_byte_2) -> Bus Creator1/3
  ESS_Manager/4(Diag_Rq_Fktnl_Data_OBD_byte_3) -> Bus Creator1/4
  ESS_Manager/5(Diag_Rq_Fktnl_Data_OBD_byte_4) -> Bus Creator1/5
  ESS_Manager/6(Diag_Rq_Fktnl_Data_OBD_byte_5) -> Bus Creator1/6
  ESS_Manager/7(Diag_Rq_Fktnl_Data_OBD_byte_6) -> Bus Creator1/7
  ESS_Manager/8(Diag_Rq_Fktnl_Data_OBD_byte_7) -> Bus Creator1/8
  ESS_Manager/10(MO_SleepAckn) -> Bus Creator2/1
  ESS_Manager/12(T_15) -> Bus Creator4/1
  Data Type Conversion6/1 -> Bus Creator3/3  "ReadyToDrive"
  Data Type Conversion7/1 -> Bus Creator3/4  "ReadyToCharge"
  Data Type Conversion8/1 -> Bus Creator3/1  "HV Discharge"
  Bus Creator1/1 -> Bus Creator/1  "ISO_Funktionaler_Req_All"
  ESS_Manager/17(HVDischarge) -> Data Type Conversion8/1
  ESS_Manager/19(ReadyToDrive) -> Data Type Conversion6/1
  ESS_Manager/20(ReadyToCharge) -> Data Type Conversion7/1
  ESS_Manager/21(Shutdown_Complete) -> Bus Creator3/5
  ESS_Manager/13(T_30) -> Bus Creator4/2
  ESS_Manager/16(chga_wake) -> Data Type Conversion1/1
  ESS_Manager/14(T_30C) -> Bus Creator4/3
  ESS_Manager/15(veh_wake) -> Bus Creator4/4
  ESS_Manager/18(HV_State) -> Bus Creator3/2
  Bus Creator3/1 -> HV_BUS_Status/1  "HV_BUS_Status"
  Controls/1 -> Bus Selector/1
  Bus Selector/1 -> ESS_Manager/19(closeMaincReq)  "<closeMaincReq>"
  Controls1/1 -> Bus Selector4/1
  Bus Creator/1 -> BMS CAN/1  "BMS_CAN"
  Bus Creator4/1 -> BMS Digital/1  "BMS_Digital"
  Data Type Conversion1/1 -> Bus Creator4/5  "chg_wake"
  Sensors/1 -> Bus Selector1/1, Bus Selector5/1, Isolation Fault Calculation/1(Sensors1), Bus Selector3/1, Bus Selector2/1
  ESS_Manager/11(MO_BMS_Sollmodus) -> Bus Creator2/2
  ESS_Manager/9(ISO_Hybrid_01_Req) -> ISO_Hybrid_01_Req/1(In1)
  ISO_Hybrid_01_Req/1(Out1) -> Bus Creator/2

== system Milford/Controller_with_Transmission_Manager1/HSC/Powertrain Manager/HV Manager1/DCDC Manager ==
  BMSInput : Inport
  In1 : Inport  Port=2
  In2 : Inport  Port=3
  Bus Creator : BusCreator  Inputs=6
  Bus Selector1 : BusSelector  OutputSignals=from_CAN.fromHV_CAN.from_BMSHybrid.BMS_HYB_02.BMS_IstModus
  Bus Selector2 : BusSelector  OutputSignals=EngOnReq,powerMode
  Bus Selector3 : BusSelector  OutputSignals=HV_req
  Chart : Stateflow chart  RequirementInfo={} %GIDa_d26a8659_2f91_4e0f_9a85_a466cd76580c  TreatAsAtomicUnit=on
  Constant : Constant  Value=3
  Contactors status check : Subsystem  Commented=on
  DCDCOVrrdSwitch : Constant  Value=0
  DCDCOVrrdVal : Constant  Value=0
  Switch : Switch  Criteria=u2 > Threshold
  Out1 : Outport
  wires:
  Bus Selector3/1 -> Chart/2(CloseMainC)  "<HV_req>"
  In2/1 -> Bus Selector3/1
  Bus Selector2/1 -> Chart/4(EngOnReq)  "<EngOnReq>"
  Bus Selector1/1 -> Chart/1(BMS_IstModus)  "<BMS_IstModus>"
  Bus Selector2/2 -> Chart/5(powerMode)  "<powerMode>"
  In1/1 -> Bus Selector2/1
  DCDCOVrrdVal/1 -> Switch/1
  DCDCOVrrdSwitch/1 -> Switch/2
  Chart/1(DCmode) -> Switch/3  "DC_mode"
  Chart/6(DCDC_State) -> Bus Creator/6  "DCDC_State"
  Bus Creator/1 -> Out1/1  "DCDC_Out"
  Chart/2(VoltageHV) -> Bus Creator/2  "VoltageHV"
  Chart/3(CurrentHV) -> Bus Creator/3  "CurrentHV"
  Chart/4(VoltageLV) -> Bus Creator/4  "VoltageLV"
  Chart/5(CurrentLV) -> Bus Creator/5  "CurrentLV"
  Switch/1 -> Bus Creator/1  "DC_mode"
  Constant/1 -> Chart/3(INV_state)
  BMSInput/1 -> Bus Selector1/1

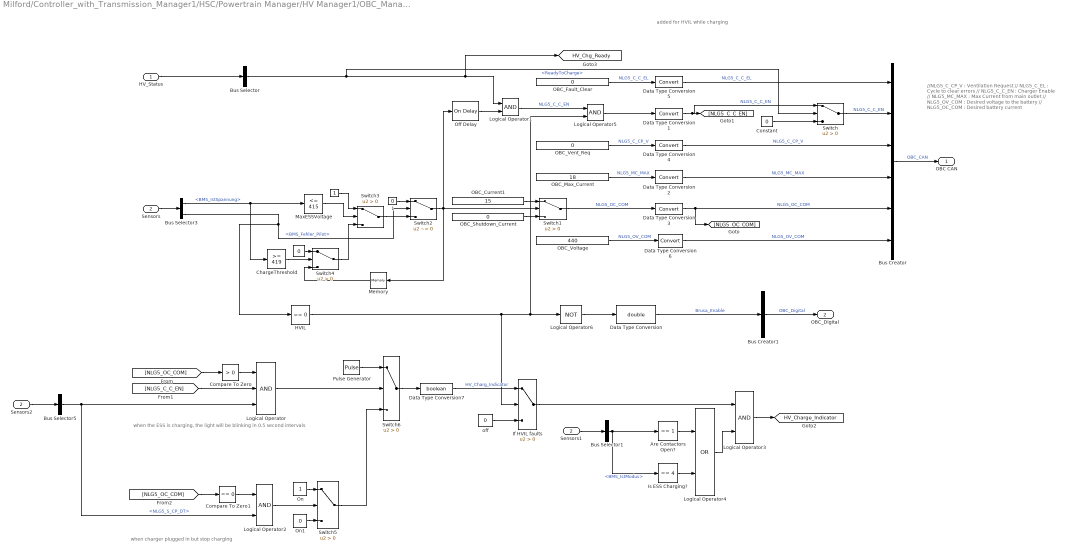
== system Milford/Controller_with_Transmission_Manager1/HSC/Powertrain Manager/HV Manager1/OBC_Manager ==
  note: when the ESS is charging, the light will be blinking in 0.5 second intervals
  note: when charger plugged in but stop charging
  note: //NLG5_C_CP_V : Ventilation Request
      | // NLG5_C_EL : Cycle to clear errors
      | // NLG5_C_C_EN : Charger Enable
      | // NLG5_MC_MAX : Max Current from main outlet
      | // NLG5_OV_COM : Desired voltage to the battery
      | // NLG5_OC_COM : Desired battery current
  note: added for HVIL
      | while charging
  HV_Status : Inport
  Sensors : Inport  Port=2
  " " : Constant
  "   " : Constant  Value=0
  "   1" : Constant  Value=0
  Are Contactors Open? : simulink/Logic and Bit Operations/Compare To Constant  relop===  const=1  OutDataTypeStr=boolean
      link override Compare: Operator===  OutDataTypeStr=boolean
  Bus Creator : BusCreator  Inputs=6
  Bus Creator1 : BusCreator  Inputs=1
  Bus Selector : BusSelector  OutputSignals=ReadyToCharge
  Bus Selector1 : BusSelector  OutputSignals=from_CAN.fromHV_CAN.from_BMSHybrid.BMS_HYB_02.BMS_IstModus
  Bus Selector3 : BusSelector  OutputSignals=from_CAN.fromHV_CAN.from_BMSHybrid.BMS_HYB_02.BMS_IstSpannung,from_CAN.fromHV_CAN.from_BMSHybrid.BMS_HYB_02.BMS_Fehler_Pilot
  Bus Selector5 : BusSelector  OutputSignals=from_CAN.fromHV_CAN.from_OBC.NLG5_ST.NLG5_S_CP_DT
  ChargeThreshold : simulink/Logic and Bit Operations/Compare To Constant  relop=>=  const=419  OutDataTypeStr=boolean
      link override Compare: Operator=>=  OutDataTypeStr=boolean
  Compare To Zero : simulink/Logic and Bit Operations/Compare To Zero  relop=>  OutDataTypeStr=boolean
      link override Compare: Operator=>  OutDataTypeStr=boolean
  Compare To Zero1 : simulink/Logic and Bit Operations/Compare To Zero  relop===  OutDataTypeStr=boolean
      link override Compare: Operator===  OutDataTypeStr=boolean
  Constant : Constant  Value=0
  Data Type Conversion : DataTypeConversion  OutDataTypeStr=double
  Data Type Conversion{1..6} (6 alike) : DataTypeConversion
  Data Type Conversion7 : DataTypeConversion  OutDataTypeStr=boolean
  HVIL : simulink/Logic and Bit Operations/Compare To Constant  relop===  const=0  OutDataTypeStr=boolean
      link override Compare: Operator===  OutDataTypeStr=boolean
  If HVIL faults : Switch  Criteria=u2 > Threshold
  Is ESS Charging? : simulink/Logic and Bit Operations/Compare To Constant  relop===  const=4  OutDataTypeStr=boolean
      link override Compare: Operator===  OutDataTypeStr=boolean
  Logical Operator : Logic  Inputs=3  AllPortsSameDT=off  OutDataTypeStr=boolean
  Logical Operator{1..3,5} (4 alike) : Logic  AllPortsSameDT=off  OutDataTypeStr=boolean
  Logical Operator4 : Logic  Operator=OR  AllPortsSameDT=off  OutDataTypeStr=boolean
  Logical Operator6 : Logic  Operator=NOT  Inputs=3  AllPortsSameDT=off  OutDataTypeStr=boolean
  MaxESSVoltage : simulink/Logic and Bit Operations/Compare To Constant  relop=<=  const=415  OutDataTypeStr=boolean
      link override Compare: Operator=<=  OutDataTypeStr=boolean
  Memory : Memory  InheritSampleTime=on
  OBC_Current1 : Constant  Value=15
  OBC_Fault_Clear : Constant  Value=0
  OBC_Max_Current : Constant  Value=18
  OBC_Shutdown_Current : Constant  Value=0
  OBC_Vent_Req : Constant  Value=0
  OBC_Voltage : Constant  Value=440
  Off Delay : powerlib_meascontrol/Logic/On Delay  DelayType=Off delay  delay=30  ic=0  Ts=0
      settings: SourceProductName=Simscape Power Systems
  On : Constant
  On1 : Constant  Value=0
  Pulse Generator : DiscretePulseGenerator  PulseType=Time based  Period=1  PulseWidth=50
  Sensors1 : InportShadow  Port=2
  Sensors2 : InportShadow  Port=2
  Switch{,1,3..6} (6 alike) : Switch  Criteria=u2 > Threshold
  Switch2 : Switch  Criteria=u2 ~= 0
  off : Constant  Value=0
  OBC CAN : Outport
  OBC_Digital : Outport  Port=2
  tag scope: HV_Charge_Indicator=global, HV_Chg_Ready=global
  wires:
  Sensors2/1 -> Bus Selector5/1
  Bus Selector5/1 -> Logical Operator/3, Logical Operator2/2  "<NLG5_S_CP_DT>"
  Switch/1 -> Bus Creator/2  "NLG5_C_C_EN"
  Constant/1 -> Switch/3
  Logical Operator6/1 -> Data Type Conversion/1
  Logical Operator5/1 -> Data Type Conversion1/1
  Logical Operator4/1 -> Logical Operator3/2
  Is ESS Charging?/1 -> Logical Operator4/2
  Bus Selector1/1 -> Are Contactors Open?/1, Is ESS Charging?/1  "<BMS_IstModus>"
  Are Contactors Open?/1 -> Logical Operator4/1
  Sensors1/1 -> Bus Selector1/1
  Logical Operator3/1 -> [HV_Charge_Indicator]
  off/1 -> If HVIL faults/3
  If HVIL faults/1 -> Logical Operator3/1
  HVIL/1 -> If HVIL faults/2, Logical Operator6/1, Logical Operator5/2
  "   1"/1 -> Switch2/1
  Switch3/1 -> Switch2/3
  Bus Creator1/1 -> OBC_Digital/1  "OBC_Digital"
  Data Type Conversion/1 -> Bus Creator1/1  "Brusa_Enable"
  Bus Selector3/2 -> Switch2/2, HVIL/1  "<BMS_Fehler_Pilot>"
  Switch6/1 -> Data Type Conversion7/1
  Switch5/1 -> Switch6/3
  On1/1 -> Switch5/3
  On/1 -> Switch5/1
  Logical Operator2/1 -> Switch5/2
  Compare To Zero1/1 -> Logical Operator2/1
  [NLG5_OC_COM] -> Compare To Zero1/1
  Pulse Generator/1 -> Switch6/1
  Logical Operator/1 -> Switch6/2
  [NLG5_C_C_EN] -> Logical Operator/2
  Compare To Zero/1 -> Logical Operator/1
  [NLG5_OC_COM] -> Compare To Zero/1
  Sensors/1 -> Bus Selector3/1
  Bus Creator/1 -> OBC CAN/1  "OBC_CAN"
  HV_Status/1 -> Bus Selector/1
  MaxESSVoltage/1 -> Switch3/2
  Bus Selector/1 -> [HV_Chg_Ready], Logical Operator1/1, Switch/2  "<ReadyToCharge>"
  Off Delay/1 -> Logical Operator1/2
  Bus Selector3/1 -> MaxESSVoltage/1, ChargeThreshold/1  "<BMS_IstSpannung>"
  Data Type Conversion2/1 -> Bus Creator/4  "NLG5_MC_MAX"
  Data Type Conversion5/1 -> Bus Creator/1  "NLG5_C_C_EL"
  Data Type Conversion4/1 -> Bus Creator/3  "NLG5_C_CP_V"
  Data Type Conversion6/1 -> Bus Creator/6  "NLG5_OV_COM"
  Data Type Conversion3/1 -> [NLG5_OC_COM], Bus Creator/5  "NLG5_OC_COM"
  OBC_Current1/1 -> Switch1/1
  Switch2/1 -> Switch1/2, Off Delay/1, Memory/1
  "   "/1 -> Switch4/1
  ChargeThreshold/1 -> Switch4/2
  " "/1 -> Switch3/1
  OBC_Shutdown_Current/1 -> Switch1/3
  Memory/1 -> Switch4/3
  Switch4/1 -> Switch3/3
  Data Type Conversion1/1 -> [NLG5_C_C_EN], Switch/1  "NLG5_C_C_EN"
  Logical Operator1/1 -> Logical Operator5/1  "NLG5_C_C_EN"
  Switch1/1 -> Data Type Conversion3/1  "NLG5_OC_COM"
  OBC_Vent_Req/1 -> Data Type Conversion4/1  "NLG5_C_CP_V"
  OBC_Fault_Clear/1 -> Data Type Conversion5/1  "NLG5_C_C_EL"
  OBC_Max_Current/1 -> Data Type Conversion2/1  "NLG5_MC_MAX"
  OBC_Voltage/1 -> Data Type Conversion6/1  "NLG5_OV_COM"
  Data Type Conversion7/1 -> If HVIL faults/1  "HV_Charg_Indicator"

== system Milford/Controller_with_Transmission_Manager1/HSC/Powertrain Manager/Torque Distribution/AxlTrq_to_EngTrq ==
  note: check this rate limiter
  note: //From engine axle torque to engine torque//
  In1 : Inport
  Compare To Constant : simulink/Logic and Bit Operations/Compare To Constant  relop===  const=0  OutDataTypeStr=boolean
  Constant1 : Constant  Value=max(gb.plant.init.ratio.map)
  Constant5 : Constant  Value=fd.plant.init.ratio
  Divide1 : Product  Inputs=*//
  Ground : Ground  Commented=on
  Rate Limiter : RateLimiter  RisingSlewLimit=1000  FallingSlewLimit=-2000
  Rate Limiter1 : RateLimiter  Commented=on  RisingSlewLimit=Engine.trq_uprate  FallingSlewLimit=Engine.trq_derate
  Ratio Filter : Subsystem
  Switch : Switch  Criteria=u2 > Threshold
  Terminator : Terminator  Commented=on
  Out1 : Outport
  wires:
  In1/1 -> Divide1/1
  Constant5/1 -> Divide1/2
  Divide1/1 -> Rate Limiter/1
  [TransRatio] -> Ratio Filter/1(Ratio)
  Compare To Constant/1 -> Switch/2
  Constant1/1 -> Switch/1
  Switch/1 -> Divide1/3
  Rate Limiter/1 -> Out1/1
  Ratio Filter/1(Filtered_Ratio) -> Switch/3, Compare To Constant/1
  Rate Limiter1/1 -> Terminator/1
  Ground/1 -> Rate Limiter1/1

== system Milford/Controller_with_Transmission_Manager1/HSC/Powertrain Manager/Torque Distribution/AxlTrq_to_MotTrq ==
  In1 : Inport
  AxlTrq_to_MtrTrq2 : Subsystem
  MotTrqLimit : Saturate  UpperLimit=250  LowerLimit=-200
  Scope : Scope  NumInputPorts=4
  Subsystem : Subsystem
  electric machine filter : Subsystem
  Out1 : Outport
  wires:
  In1/1 -> AxlTrq_to_MtrTrq2/1(In1)
  AxlTrq_to_MtrTrq2/1(MtrTrqCmd) -> Scope/1, electric machine filter/1(trq)  "MtrTrqCmd"
  electric machine filter/1(filtered) -> Scope/2, MotTrqLimit/1  "MtrTrqCmd"
  Subsystem/1(Out1) -> Scope/4, Out1/1  "MtrTrqCmd"
  MotTrqLimit/1 -> Scope/3, Subsystem/1(In1)  "MtrTrqCmd"
  [MotorSpeed] -> Subsystem/2(RPM)

== system Milford/Controller_with_Transmission_Manager1/HSC/Powertrain Manager/Torque Distribution/Engine Trq Limit ==
  In1 : Inport
  EngTrqMismchDegraded : Inport  Port=2
  EngTrqMismchLimp : Inport  Port=3
  Eng_TempRange : Inport  Port=4
  iceSystemStatus : Inport  Port=5
  Compare To Constant : simulink/Logic and Bit Operations/Compare To Constant  relop===  const=1  OutDataTypeStr=boolean
  Eng Troque Mismatch Mitigation : Subsystem
  OverTemperature Mitigation : Subsystem
  Switch2 : Switch  Threshold=1
  Out1 : Outport
  wires:
  Switch2/1 -> Out1/1
  Compare To Constant/1 -> Switch2/2
  EngTrqMismchLimp/1 -> Eng Troque Mismatch Mitigation/3(EngTrqMismchLimp)
  EngTrqMismchDegraded/1 -> Eng Troque Mismatch Mitigation/2(EngTrqMismchDegraded)
  Eng_TempRange/1 -> OverTemperature Mitigation/2(essTempRange)
  Eng Troque Mismatch Mitigation/1(Out1) -> OverTemperature Mitigation/1(In1)
  In1/1 -> Eng Troque Mismatch Mitigation/1(In1), Switch2/3
  iceSystemStatus/1 -> Compare To Constant/1
  OverTemperature Mitigation/1(Out1) -> Switch2/1

== system Milford/Controller_with_Transmission_Manager1/HSC/Powertrain Manager/Torque Distribution/Motor Troque Mismatch Mitigation_CD ==
  In1 : Inport
  MotTrqMismchDegraded : Inport  Port=2
  MotTrqMismchLimp : Inport  Port=3
  Subsystem : Subsystem
  Out1 : Outport
  tag scope: TorqueRequest_Nm=global
  wires:
  In1/1 -> [TorqueRequest_Nm]
  MotTrqMismchLimp/1 -> Subsystem/1(In1)
  MotTrqMismchDegraded/1 -> Subsystem/2(In2)
  Subsystem/1(Out1) -> Out1/1

== system Milford/Controller_with_Transmission_Manager1/HSC/Powertrain Manager/Torque Distribution/OverTemperature Mitigation_CD ==
  In1 : Inport
  essTempRange : Inport  Port=2
  MCUTempRange : Inport  Port=3
  MotorTempRange : Inport  Port=4
  Compare To Constant : simulink/Logic and Bit Operations/Compare To Constant  relop===  const=1  OutDataTypeStr=boolean
  Compare To Constant1 : simulink/Logic and Bit Operations/Compare To Constant  relop===  const=3  OutDataTypeStr=boolean
  Compare To Constant2 : simulink/Logic and Bit Operations/Compare To Constant  relop===  const=1  OutDataTypeStr=boolean
  Compare To Constant3 : simulink/Logic and Bit Operations/Compare To Constant  relop===  const=3  OutDataTypeStr=boolean
  Compare To Constant4 : simulink/Logic and Bit Operations/Compare To Constant  relop===  const=1  OutDataTypeStr=boolean
  Compare To Constant5 : simulink/Logic and Bit Operations/Compare To Constant  relop===  const=3  OutDataTypeStr=boolean
  Constant3 : Constant  Value=mot.plant.init.trq_posmax
  Constant5 : Constant  Value=mot.plant.init.trq_posmax
  Gain1 : Gain  Gain=0.4
  Gain3 : Gain  Gain=0.5
  Logical Operator : Logic  Operator=OR  AllPortsSameDT=off  OutDataTypeStr=boolean
  Logical Operator1 : Logic  Operator=OR  AllPortsSameDT=off  OutDataTypeStr=boolean
  Logical Operator2 : Logic  Operator=OR  AllPortsSameDT=off  OutDataTypeStr=boolean
  MinMax1 : MinMax  Inputs=2
  MinMax2 : MinMax  Inputs=2
  Switch1 : Switch  Threshold=1
  Switch2 : Switch  Threshold=1
  Switch3 : Switch  Threshold=1
  Out1 : Outport
  wires:
  MotorTempRange/1 -> Compare To Constant5/1, Compare To Constant4/1
  Constant5/1 -> Gain3/1
  Logical Operator1/1 -> Switch2/2
  Compare To Constant1/1 -> Logical Operator/2
  Compare To Constant/1 -> Logical Operator/1
  Constant3/1 -> Gain1/1
  MinMax2/1 -> Switch3/1, Switch2/1
  MinMax1/1 -> Switch1/1
  Logical Operator/1 -> Switch1/2
  Logical Operator2/1 -> Switch3/2
  In1/1 -> MinMax2/1, Switch1/3, MinMax1/1
  Gain1/1 -> MinMax2/2
  Gain3/1 -> MinMax1/2
  Switch2/1 -> Switch3/3
  MCUTempRange/1 -> Compare To Constant3/1, Compare To Constant2/1
  Compare To Constant2/1 -> Logical Operator1/1
  Compare To Constant3/1 -> Logical Operator1/2
  essTempRange/1 -> Compare To Constant1/1, Compare To Constant/1
  Switch1/1 -> Switch2/3
  Compare To Constant4/1 -> Logical Operator2/1
  Compare To Constant5/1 -> Logical Operator2/2
  Switch3/1 -> Out1/1

== system Milford/Controller_with_Transmission_Manager1/HSC/Powertrain Manager/Torque Distribution/Select_APP ==
  APP_Select : Constant  Value=0
  Data Type Conversion10 : DataTypeConversion  OutDataTypeStr=boolean
  Switch1 : Switch  Criteria=u2 > Threshold
  EngAppReq : Outport
  wires:
  Switch1/1 -> EngAppReq/1  "EngAppReq"
  APP_Select/1 -> Data Type Conversion10/1
  Data Type Conversion10/1 -> Switch1/2
  [AccPos_Perc] -> Switch1/1
  [EngAppReq] -> Switch1/3

== system Milford/Controller_with_Transmission_Manager1/HSC/Powertrain Manager/Torque Distribution/Sport Mode Enable ==
  In1 : Inport
  Bus Selector5 : BusSelector  OutputSignals=from_Analog.Sport_Mode_SW
  Compare To Constant : simulink/Logic and Bit Operations/Compare To Constant  relop===  const=2  OutDataTypeStr=boolean
  Sports Mode Logic : Stateflow chart  TreatAsAtomicUnit=on
  Out1 : Outport
  wires:
  Compare To Constant/1 -> Out1/1
  Sports Mode Logic/1(Driver_Mode) -> Compare To Constant/1
  Bus Selector5/1 -> Sports Mode Logic/1(Voltage_Input)  "<Sport_Mode_SW>"
  In1/1 -> Bus Selector5/1

== system Milford/Controller_with_Transmission_Manager1/HSC/Powertrain Manager/Torque Distribution/Subsystem1 ==
  SoC : Inport
  CS_On : Inport  Port=2
  Constant : Constant
  Sample and Hold1 : dspsigops/Sample and Hold  trig=Rising edge  initCond=0  latchinput=off
  Switch : Switch  Criteria=u2 > Threshold
  Faked_SoC : Outport
  wires:
  Constant/1 -> Switch/3
  Sample and Hold1/1 -> Switch/1
  Switch/1 -> Faked_SoC/1
  CS_On/1 -> Sample and Hold1/Trigger, Switch/2
  SoC/1 -> Sample and Hold1/1

== system Milford/Controller_with_Transmission_Manager1/HSC/Powertrain Manager/Torque Distribution/Supervisory  Control  Logic1/VehReady.CD_Mode.Brake_mode.MotTrqCalc1 ==
  note: Regenerative braking:
      | Regenerative braking should be allowed under specific chassis speed:
      | chas_spd_below_no_regen= 1.5;
      | chas_spd_above_full_regen = 3;
      | ess_soc_above_regen_forbidden = .92;  % ESS SOC above which regen braking is forbidden
      | ess_soc_above_regen_allowed = .9;% ESS SOC above which regen braking is allowed
  BPP : Inport
  VehSpd : Inport  Port=2
  ShftLvrPos : Inport  Port=3
  MotSpeed : Inport  Port=4
  TransRatio : Inport  Port=5
  IntdAxleTrq : Inport  Port=6
  f : TriggerPort  TriggerType=function-call  VariantControl=Variant
      settings: CopyFcn=Stateflow.SLINSF.SimulinkMan.removeBlockPreDeleteFcn  PreDeleteFcn=Stateflow.SLINSF.SimulinkMan.unsafePredeleteFcn
  "% to 1 " : Gain  Gain=1/100
  Constant : Constant  Value=0
  Constant1 : Constant  Value=0
  Constant2 : Constant  Value=fd.plant.init.ratio
  Divide : Product  Inputs=***
  Divide2 : Product  Inputs=***
  Index Vector : MultiPortSwitch  DataPortOrder=Zero-based contiguous  Inputs=5  zeroidx=on
  MinMax : MinMax  Function=max  Inputs=2
  Peak trq max - Regen : Lookup  InputValues=mot.plant.init.regen.trq_max.idx1_spd  Table=mot.plant.init.regen.trq_max.map  LookUpMeth=Interpolation-Use End Values  SaturateOnIntegerOverflow=on
  Regen Trq Derating1 : Lookup_n-D  Commented=on  NumberOfTableDimensions=1  BreakpointsForDimension1=[0 10 20 30 40]  Table=[0 0.025 0.05 0.1 1]  ExtrapMethod=Clip  UseLastTableValue=on  InternalRulePriority=Speed  RndMeth=Simplest  InputSameDT=on
  Regen Trq Derating2 : Lookup_n-D  NumberOfTableDimensions=1  BreakpointsForDimension1=[0 10 11 200]  Table=[0 0.5 1 1]  ExtrapMethod=Clip  UseLastTableValue=on  InternalRulePriority=Speed  RndMeth=Simplest  InputSameDT=on
  Regen_derat_overri : Constant  Value=0
  Regen_derat_value : Constant  Value=0.5
  Switch : Switch  Criteria=u2 > Threshold
  limit to -200Nm : Saturate  UpperLimit=0  LowerLimit=-200
  T : Outport
  wires:
  BPP/1 -> "% to 1 "/1
  "% to 1 "/1 -> Divide/1
  Divide/1 -> limit to -200Nm/1
  VehSpd/1 -> Regen Trq Derating2/1
  ShftLvrPos/1 -> Index Vector/1
  [TrqCalc] -> Index Vector/4  "R"
  [TrqCalc] -> Index Vector/6  "D"
  Index Vector/1 -> T/1
  Constant/1 -> Index Vector/2  "Between Ranges"
  Constant1/1 -> Index Vector/3  "P"
  [TrqCalc] -> Index Vector/5  "N"
  MotSpeed/1 -> Peak trq max - Regen/1  "RPM"
  Peak trq max - Regen/1 -> Divide/2
  Constant2/1 -> Divide2/1
  limit to -200Nm/1 -> Divide2/2
  TransRatio/1 -> Divide2/3
  Divide2/1 -> MinMax/2  "motor"
  Regen Trq Derating2/1 -> Switch/3
  Regen_derat_overri/1 -> Switch/2
  Switch/1 -> Divide/3
  Regen_derat_value/1 -> Switch/1
  IntdAxleTrq/1 -> MinMax/1
  MinMax/1 -> [TrqCalc]

== system Milford/Controller_with_Transmission_Manager1/HSC/Powertrain Manager/Torque Distribution/Supervisory  Control  Logic1/VehReady.CD_Mode.Brake_mode.MotTrqCalc2 ==
  note: Regenerative braking:
      | Regenerative braking should be allowed under specific chassis speed:
      | chas_spd_below_no_regen= 1.5;
      | chas_spd_above_full_regen = 3;
      | ess_soc_above_regen_forbidden = .92;  % ESS SOC above which regen braking is forbidden
      | ess_soc_above_regen_allowed = .9;% ESS SOC above which regen braking is allowed
  ShftLvrPos : Inport
  TransRatio : Inport  Port=2
  f : TriggerPort  TriggerType=function-call  VariantControl=Variant
      settings: CopyFcn=Stateflow.SLINSF.SimulinkMan.removeBlockPreDeleteFcn  PreDeleteFcn=Stateflow.SLINSF.SimulinkMan.unsafePredeleteFcn
  Constant : Constant  Value=0
  Constant1 : Constant  Value=0
  Constant2 : Constant  Value=fd.plant.init.ratio
  Divide2 : Product  Inputs=***
  Idle_torque_Regen : Constant  Value=0
  Index Vector : MultiPortSwitch  DataPortOrder=Zero-based contiguous  Inputs=5  zeroidx=on
  T : Outport
  wires:
  ShftLvrPos/1 -> Index Vector/1
  [TrqCalc] -> Index Vector/4  "R"
  [TrqCalc] -> Index Vector/6  "D"
  Index Vector/1 -> T/1
  Constant/1 -> Index Vector/2  "Between Ranges"
  Constant1/1 -> Index Vector/3  "P"
  [TrqCalc] -> Index Vector/5  "N"
  Constant2/1 -> Divide2/1
  TransRatio/1 -> Divide2/3
  Divide2/1 -> [TrqCalc]  "motor"
  Idle_torque_Regen/1 -> Divide2/2
